simulink model "Component"  (R2013a)
settings: Solver=ode45  StartTime=0.0  StopTime=10.0  RelTol=1e-3
settings Model: Creator=sz609516  LastModifiedBy=sz609516

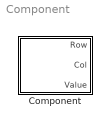
== system Component ==
  Component : Subsystem

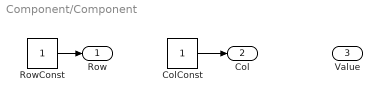
== system Component/Component ==
  ColConst : Constant
  RowConst : Constant
  Row : Outport
  Col : Outport  Port=2
  Value : Outport  Port=3
  wires:
  RowConst/1 -> Row/1
  ColConst/1 -> Col/1
